simulink model "PMSM_New_MTPA"  (R2018b)
settings: Solver=ode45  StartTime=0.0  StopTime=15  FixedStep=Ts  RelTol=1e-4  EnableMultiTasking=on
InitFcn:
  | Ts = 1e-4;
  | 
  | 
  | Rs = 0.8975;
  | Ld = 15e-3;
  | Lq = 19e-3;
  | Pn = 3;
  | flux = 0.1764;
  | 
  | kp_comp = 0.65;
  | ki_comp = 0.001*pi*kp_comp;
  | 
  | kp_FW = 1;
  | ki_FW = 0;
undefined symbols (not defined in the file or in its folder): DiscIntNeverNeededParam
libraries: powerlib x5, powerlib_extras x2, simulink x1
settings Model: Creator=SUN  LastModifiedBy=liangjin
settings SolverCC: ZeroCrossControl=DisableAll
settings DataIOCC: LimitDataPoints=on  SaveFormat=Array
settings OptimizationCC: ExpressionDepthLimit=2147483647  InitFltsAndDblsToZero=on  LifeSpan=inf
settings DebuggingCC: UnderspecifiedInitializationDetection=Classic  MergeDetectMultiDrivingBlocksExec=none  SolverPrmCheckMsg=warning  FcnCallInpInsideContextMsg=warning  StateNameClashWarn=warning  SFUnexpectedBacktrackingDiag=warning  SFNoUnconditionalDefaultTransitionDiag=warning  SFExecutionAtInitializationDiag=none
settings HardwareCC: ProdBitPerPointer=32  ProdBitPerSizeT=32  ProdBitPerPtrDiffT=32  ProdLargestAtomicFloat=None  ProdIntDivRoundTo=Undefined  ProdEndianess=Unspecified  ProdWordSize=32  ProdHWDeviceType=32-bit Generic
settings ModelReferenceCC: PropagateSignalLabelsOutOfModel=off
settings SFSimCC: SimUseLocalCustomCode=off
settings RTWCC: RTWUseLocalCustomCode=off
settings CodeAppCC: StateflowObjectComments=on
settings GRTTargetCC: TargetLangStandard=C89/C90 (ANSI)  GeneratePreprocessorConditionals=Disable all  CombineOutputUpdateFcns=off  GRTInterface=on
settings ConfigComp: CovMetricSettings=dw  CovHtmlReporting=on  CovSaveCumulativeToWorkspaceVar=on  CovSaveSingleToWorkspaceVar=on  CovExternalEMLEnable=off  CovSFcnEnable=off
settings SimscapeCC: SimscapeNormalizeSystem=off

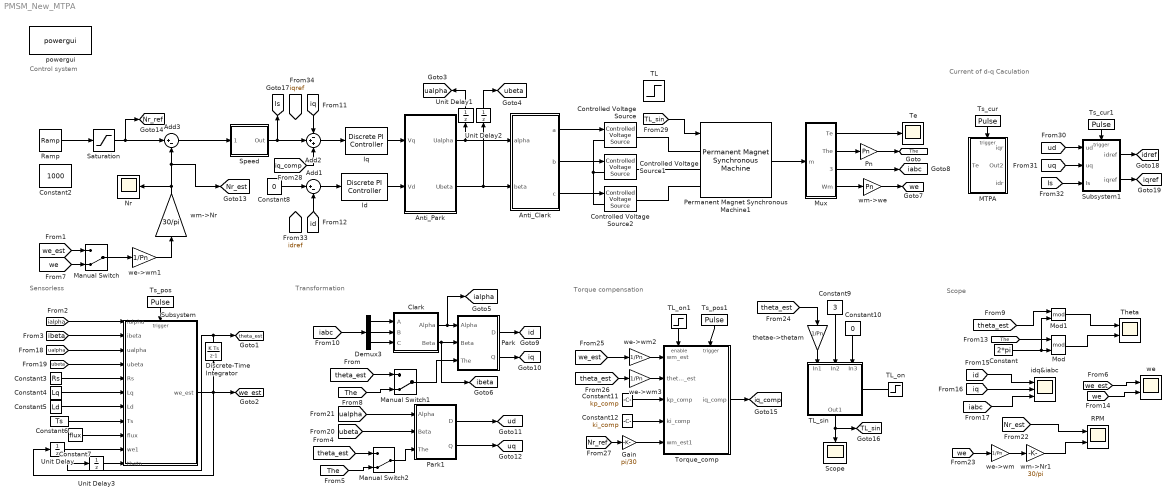
== system PMSM_New_MTPA ==
  note: Torque compensation
  note: Scope
  note: Control system
  note: Transformation
  note: Sensorless
  note: Current of d-q Caculation
  Add1 : Sum  Inputs=|+-
  Add2 : Sum  Inputs=-++
  Add3 : Sum  Inputs=|+-
  Anti_Clark : Subsystem
  Anti_Park : Subsystem
  Clark : Subsystem
  Constant : Constant  Value=2*pi
  Constant10 : Constant  Value=0
  Constant11 : Constant  Value=kp_comp
  Constant12 : Constant  Value=ki_comp
  Constant2 : Constant  Value=1000
  Constant3 : Constant  Value=Rs
  Constant4 : Constant  Value=Lq
  Constant5 : Constant  Value=Ld
  Constant6 : Constant  Value=Ts
  Constant7 : Constant  Value=flux
  Constant8 : Constant  Value=0
  Constant9 : Constant  Value=3
  Controlled Voltage Source : powerlib/Electrical Sources/Controlled Voltage Source  Initialize=on  Source_Type=AC  Amplitude=0  Phase=0  Frequency=0  Measurements=Voltage
      settings: SourceProductName=Simscape Electrical
  Controlled Voltage Source1 : powerlib/Electrical Sources/Controlled Voltage Source  Initialize=on  Source_Type=AC  Amplitude=0  Phase=0  Frequency=0  Measurements=Voltage
      settings: SourceProductName=Simscape Electrical
  Controlled Voltage Source2 : powerlib/Electrical Sources/Controlled Voltage Source  Initialize=on  Source_Type=AC  Amplitude=0  Phase=0  Frequency=0  Measurements=Voltage
      settings: SourceProductName=Simscape Electrical
  Demux3 : Demux  Outputs=3
  Discrete-Time Integrator : DiscreteIntegrator  gainval=1  SampleTime=Ts  ICPrevOutput=DiscIntNeverNeededParam  ICPrevScaledInput=DiscIntNeverNeededParam
  Gain : Gain  Gain=pi/30
  Id : powerlib_extras/Discrete  Control Blocks/Discrete PI Controller  Kp=Ld*376  Ki=Rs*376  Par_Limits=[311*sqrt(1/3) -311*sqrt(1/3)]  Init=0  Ts=Ts
  Iq : powerlib_extras/Discrete  Control Blocks/Discrete PI Controller  Kp=Lq*376  Ki=Rs*376  Par_Limits=[311*sqrt(1/3) -311*sqrt(1/3)]  Init=0  Ts=Ts
  MTPA : Subsystem
  Manual Switch : ManualSwitch  CurrentSetting=0
  Manual Switch1 : ManualSwitch  CurrentSetting=0
  Manual Switch2 : ManualSwitch  CurrentSetting=0
  Mod : Math  Operator=mod  SaturateOnIntegerOverflow=on
  Mod1 : Math  Operator=mod  SaturateOnIntegerOverflow=on
  Mux : Subsystem
  Nr : Scope
  Park : Subsystem
  Park1 : Subsystem
  Permanent Magnet Synchronous Machine1 : powerlib/Machines/Permanent Magnet Synchronous Machine  NbPhases=3  FluxDistribution=Sinusoidal  RotorType=Salient-pole  MechanicalLoad=Torque Tm  PresetModel=No  ShowDetailedParameters=on  MeasurementBus=off  Resistance=0.8975  Inductance=8.5e-3  dqInductances=[15e-3,19e-3]  La=0.000835  MachineConstant=Flux linkage established by magnets (V.s)  Flux=0.1764  VoltageCst=95.9863  TorqueCst=0.7938  Flat=120  Mechanical=[0.000311 0.0000001 3]  PolePairs=3  InitialConditions=[0,0, 0,0]  InitialConditions5ph=[0 0 0 0 0 0]  TsPowergui=0  TsBlock=Ts  RefAngle=Aligned with phase A axis (original Park)
  Pn : Gain  Gain=Pn
  RPM : Scope  NumInputPorts=2
  Ramp : simulink/Sources/Ramp  slope=250  start=0  InitialOutput=0
  Saturation : Saturate  UpperLimit=1000  LowerLimit=-1000
  Scope : Scope
  Speed : Subsystem  AncestorBlock=|  DialogController=POWERSYS.PowerSysDialog  mask(Discrete PI Controller){Kpw=0.01, Kiw=0.01*50, Ba=0, Par_Limits=[50 -50], Init=0, Ts=Ts}
      | powerlib_extras/Discrete 
      | Control Blocks/Discrete
      | PI Controller
      mask prompts: Kpw "Proportional gain (Kp):"; Kiw "Integral gain (Ki):"; Ba "feedback gain (Ba)"; Par_Limits "Output limits: [ Upper   Lower ]"; Init "Output initial value:"; Ts "Sample time:"
      mask help: This block implements a discrete PI controller.
      mask init:
      | UpperLimit=Par_Limits(1);
      | LowerLimit=Par_Limits(2);
      | power_initmask();
      mask Help: This block is part of a subset of blocks in the Extras library that does not have documentation associated with it, other than the block mask description.
      mask Display: disp('PI');
  Subsystem : Subsystem
  Subsystem1 : Subsystem
  TL : Step  Time=5  After=7  SampleTime=Ts
  TL_on : Step  Time=5  SampleTime=0
  TL_on1 : Step  Time=5  SampleTime=0
  TL_sin : Subsystem
  Te : Scope
  Theta : Scope  NumInputPorts=2
  Torque_comp : Subsystem
  Ts_cur : DiscretePulseGenerator  PulseType=Time based  Period=Ts  PulseWidth=50
  Ts_cur1 : DiscretePulseGenerator  PulseType=Time based  Period=Ts  PulseWidth=50
  Ts_pos : DiscretePulseGenerator  PulseType=Time based  Period=Ts  PulseWidth=50
  Ts_pos1 : DiscretePulseGenerator  PulseType=Time based  Period=Ts  PulseWidth=50
  Unit Delay{,1..3} (4 alike) : UnitDelay  SampleTime=Ts
  idq&iabc : Scope  NumInputPorts=3
  powergui : powerlib/powergui  SimulationMode=Discrete  SampleTime=1e-5  frequency=60  Iterations=50  frequencyindice=0  Pbase=100e6  ErrMax=1e-4  UnitsV=kV  UnitsW=MW  buscounter=0  FunctionMessages=off  echomessages=off  EnableUseOfTLC=off  CurrentSourceSwitches=off  DisableSnubberDevices=off  DisableRonSwitches=off  DisableVfSwitches=off  DisplayEquations=off  SolverType=Tustin/Backward Euler (TBE)  Interpol=off  ExternalGateDelay=off  methode=off  Ts=100  x0status=blocks  SPID=off  SwTol=0  HookPort=off  RestoreLinks=warning  ResistiveCurrentMeasurement=off  Frange=[0:2:500]  Ylog=off  Xlog=on  ShowGrid=off  save=off  variable=ZData  structure=0  ZoomFFT=on  StartTime=0.0  cycles=1  DisplayStyle=1  fundamental=60  FreqAxis=off  MaxFrequency=1000  frequencyindicesteady=1  RmsSteady=1  display=off
  thetae->thetam : Gain  Gain=1/Pn
  we : Scope  NumInputPorts=2
  we->wm{,1..3} (4 alike) : Gain  Gain=1/Pn
  wm->Nr : Gain  Gain=30/pi
  wm->Nr1 : Gain  Gain=30/pi
  wm->we : Gain  Gain=Pn
  tag scope: Is=global, Nr_est=global, Nr_ref=global, TL_sin=global, The=global, iabc=global, ialpha=global, ibeta=global, id=global, idref=global, iq=global, iq_comp=global, iqref=global, theta_est=global, ualpha=global, ubeta=global, ud=global, uq=global, we=global, we_est=global
  wires:
  Permanent Magnet Synchronous Machine1/1 -> Mux/1(m)
  Add3/1 -> Speed/1(Error)
  wm->Nr/1 -> [Nr_est], Add3/2, Nr/1
  Mux/1(Te) -> Te/1
  Mux/2(The) -> Pn/1
  Pn/1 -> [The]
  Mux/4(Wm) -> wm->we/1
  Mux/3(Iabc) -> [iabc]
  Clark/1(Alpha) -> [ialpha], Park/1(Alpha)
  Demux3/1 -> Clark/1(A)
  Demux3/2 -> Clark/2(B)
  Demux3/3 -> Clark/3(C)
  Clark/2(Beta) -> Park/2(Beta), [ibeta]
  Iq/1 -> Anti_Park/1(Vq)
  Id/1 -> Anti_Park/2(Vd)
  Anti_Clark/2(b) -> Controlled Voltage Source1/1
  Anti_Clark/3(c) -> Controlled Voltage Source2/1
  Constant/1 -> Mod1/2, Mod/2
  Mod/1 -> Theta/2
  wm->we/1 -> [we]
  Ramp/1 -> Saturation/1
  we->wm1/1 -> wm->Nr/1
  Anti_Park/1(Ualpha) -> Unit Delay1/1, Anti_Clark/1(alpha)
  Anti_Park/2(Ubeta) -> Unit Delay2/1, Anti_Clark/2(beta)
  [we_est] -> we/1
  [we_est] -> Manual Switch/1
  [we] -> Manual Switch/2
  [theta_est] -> Manual Switch1/1
  Manual Switch1/1 -> Park/3(The)
  [The] -> Manual Switch1/2
  Park/1(D) -> [id]
  Park/2(Q) -> [iq]
  [The] -> Mod/1
  [id] -> idq&iabc/1
  [iq] -> idq&iabc/2
  [iabc] -> idq&iabc/3
  [id] -> Add1/2
  [iq] -> Add2/1
  Manual Switch/1 -> we->wm1/1
  [The] -> Manual Switch2/2
  Manual Switch2/1 -> Park1/3(The)
  [theta_est] -> Manual Switch2/1
  [ubeta] -> Park1/2(Beta)
  [ualpha] -> Park1/1(Alpha)
  Park1/1(D) -> [ud]
  Park1/2(Q) -> [uq]
  Unit Delay1/1 -> [ualpha]
  Unit Delay2/1 -> [ubeta]
  Subsystem/1(we_est) -> Discrete-Time Integrator/1, [we_est], Unit Delay/1
  Constant3/1 -> Subsystem/5(Rs)
  Constant4/1 -> Subsystem/6(Lq)
  Constant5/1 -> Subsystem/7(Ld)
  Constant6/1 -> Subsystem/8(Ts)
  Constant7/1 -> Subsystem/9(flux)
  Unit Delay/1 -> Subsystem/10(we1)
  Ts_pos/1 -> Subsystem/Trigger
  Unit Delay3/1 -> Subsystem/11(theta)
  [theta_est] -> Mod1/1
  Mod1/1 -> Theta/1
  [iabc] -> Demux3/1
  Discrete-Time Integrator/1 -> [theta_est], Unit Delay3/1
  Anti_Clark/1(a) -> Controlled Voltage Source/1
  [ialpha] -> Subsystem/1(ialpha)
  [ibeta] -> Subsystem/2(ibeta)
  [ualpha] -> Subsystem/3(ualpha)
  [ubeta] -> Subsystem/4(ubeta)
  [we] -> we->wm/1
  we->wm/1 -> wm->Nr1/1
  wm->Nr1/1 -> RPM/2
  [Nr_est] -> RPM/1
  Saturation/1 -> [Nr_ref], Add3/1
  Ts_cur/1 -> MTPA/Trigger
  Add2/1 -> Iq/1
  Add1/1 -> Id/1
  [we] -> we/2
  [theta_est] -> thetae->thetam/1
  thetae->thetam/1 -> TL_sin/1(In1)
  Constant9/1 -> TL_sin/2(In2)
  Constant10/1 -> TL_sin/3(In3)
  TL_on/1 -> TL_sin/Enable
  Speed/1(Out) -> Add2/2, [Is]
  TL_sin/1(Out1) -> [TL_sin], Scope/1
  we->wm2/1 -> Torque_comp/1(wm_est)
  we->wm3/1 -> Torque_comp/2(thetam_est)
  Constant11/1 -> Torque_comp/3(kp_comp)
  Constant12/1 -> Torque_comp/4(ki_comp)
  Torque_comp/1(iq_comp) -> [iq_comp]
  [Nr_ref] -> Gain/1
  Gain/1 -> Torque_comp/5(wm_est1)
  Ts_pos1/1 -> Torque_comp/Trigger
  TL_on1/1 -> Torque_comp/Enable
  [we_est] -> we->wm2/1
  [theta_est] -> we->wm3/1
  [ud] -> Subsystem1/1(ud)
  [uq] -> Subsystem1/2(uq)
  [Is] -> Subsystem1/3(Is)
  Ts_cur1/1 -> Subsystem1/Trigger
  Subsystem1/1(idref) -> [idref]
  Subsystem1/2(iqref) -> [iqref]
  Constant8/1 -> Add1/1
  [iq_comp] -> Add2/3
  [TL_sin] -> Permanent Magnet Synchronous Machine1/1
  connections:
  Controlled Voltage Source/LConn1 -- Controlled Voltage Source2/LConn1 -- Controlled Voltage Source1/LConn1
  Controlled Voltage Source/RConn1 -- Permanent Magnet Synchronous Machine1/LConn1
  Controlled Voltage Source1/RConn1 -- Permanent Magnet Synchronous Machine1/LConn2
  Controlled Voltage Source2/RConn1 -- Permanent Magnet Synchronous Machine1/LConn3

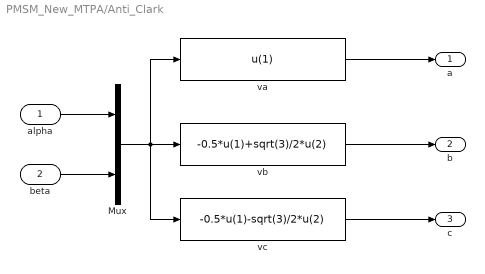
== system PMSM_New_MTPA/Anti_Clark ==
  alpha : Inport
  beta : Inport  Port=2
  Mux : Mux  Inputs=2
  va : Fcn  Expr=u(1)
  vb : Fcn  Expr=-0.5*u(1)+sqrt(3)/2*u(2)
  vc : Fcn  Expr=-0.5*u(1)-sqrt(3)/2*u(2)
  a : Outport
  b : Outport  Port=2
  c : Outport  Port=3
  wires:
  va/1 -> a/1
  beta/1 -> Mux/2
  alpha/1 -> Mux/1
  Mux/1 -> vc/1, vb/1, va/1
  vb/1 -> b/1
  vc/1 -> c/1

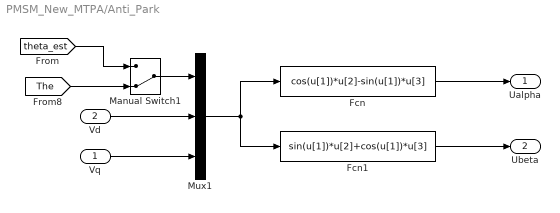
== system PMSM_New_MTPA/Anti_Park ==
  Vq : Inport
  Vd : Inport  Port=2
  Fcn : Fcn  Expr=cos(u[1])*u[2]-sin(u[1])*u[3]
  Fcn1 : Fcn  Expr=sin(u[1])*u[2]+cos(u[1])*u[3]
  Manual Switch1 : ManualSwitch  CurrentSetting=0
  Mux1 : Mux  Inputs=3
  Ualpha : Outport
  Ubeta : Outport  Port=2
  wires:
  Fcn1/1 -> Ubeta/1
  Fcn/1 -> Ualpha/1
  Mux1/1 -> Fcn/1, Fcn1/1
  Vd/1 -> Mux1/2
  Vq/1 -> Mux1/3
  Manual Switch1/1 -> Mux1/1
  [The] -> Manual Switch1/2
  [theta_est] -> Manual Switch1/1

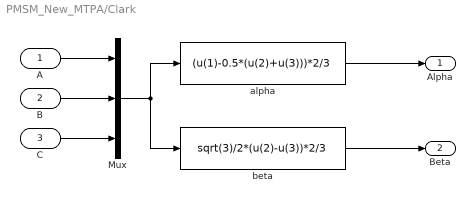
== system PMSM_New_MTPA/Clark ==
  A : Inport
  B : Inport  Port=2
  C : Inport  Port=3
  Mux : Mux  Inputs=3
  alpha : Fcn  Expr=(u(1)-0.5*(u(2)+u(3)))*2/3
  beta : Fcn  Expr=sqrt(3)/2*(u(2)-u(3))*2/3
  Alpha : Outport
  Beta : Outport  Port=2
  wires:
  alpha/1 -> Alpha/1
  B/1 -> Mux/2
  C/1 -> Mux/3
  A/1 -> Mux/1
  Mux/1 -> beta/1, alpha/1
  beta/1 -> Beta/1

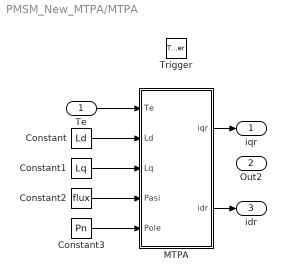
== system PMSM_New_MTPA/MTPA ==
  Te : Inport
  Trigger : TriggerPort  VariantControl=Variant  PortDimensions=1
  Constant : Constant  Value=Ld
  Constant1 : Constant  Value=Lq
  Constant2 : Constant  Value=flux
  Constant3 : Constant  Value=Pn
  MTPA : MATLAB Function  TreatAsAtomicUnit=on
  iqr : Outport
  Out2 : Outport  Port=2
  idr : Outport  Port=3
  wires:
  MTPA/2(idr) -> idr/1
  MTPA/1(iqr) -> iqr/1
  Te/1 -> MTPA/1(Te)
  Constant/1 -> MTPA/2(Ld)
  Constant1/1 -> MTPA/3(Lq)
  Constant3/1 -> MTPA/5(Pole)
  Constant2/1 -> MTPA/4(Pasi)

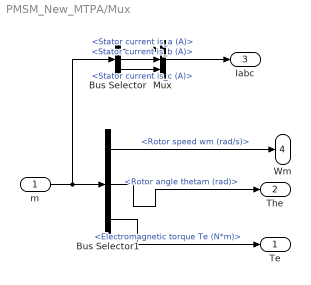
== system PMSM_New_MTPA/Mux ==
  m : Inport
  Bus Selector : BusSelector  OutputSignals=Stator current is_a (A),Stator current is_b (A),Stator current is_c (A)
  Bus Selector1 : BusSelector  OutputSignals=Rotor speed wm (rad/s),Rotor angle thetam (rad),Electromagnetic torque Te (N*m)
  Mux : Mux  Inputs=3
  Te : Outport
  The : Outport  Port=2
  Iabc : Outport  Port=3
  Wm : Outport  Port=4
  wires:
  Bus Selector1/1 -> Wm/1  "<Rotor speed wm (rad/s)>"
  Bus Selector1/2 -> The/1  "<Rotor angle thetam (rad)>"
  Bus Selector1/3 -> Te/1  "<Electromagnetic torque Te (N*m)>"
  m/1 -> Bus Selector/1, Bus Selector1/1
  Bus Selector/2 -> Mux/2  "<Stator current is_b (A)>"
  Bus Selector/3 -> Mux/3  "<Stator current is_c (A)>"
  Bus Selector/1 -> Mux/1  "<Stator current is_a (A)>"
  Mux/1 -> Iabc/1

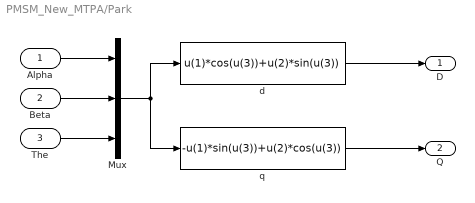
== system PMSM_New_MTPA/Park ==
  Alpha : Inport
  Beta : Inport  Port=2
  The : Inport  Port=3
  Mux : Mux  Inputs=3
  d : Fcn  Expr=u(1)*cos(u(3))+u(2)*sin(u(3))
  q : Fcn  Expr=-u(1)*sin(u(3))+u(2)*cos(u(3))
  D : Outport
  Q : Outport  Port=2
  wires:
  d/1 -> D/1
  Beta/1 -> Mux/2
  Alpha/1 -> Mux/1
  Mux/1 -> q/1, d/1
  q/1 -> Q/1
  The/1 -> Mux/3

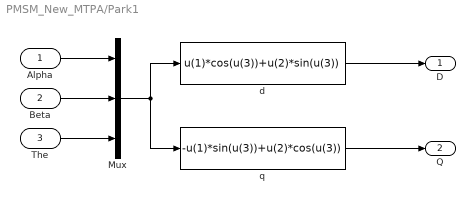
== system PMSM_New_MTPA/Park1 ==
  Alpha : Inport
  Beta : Inport  Port=2
  The : Inport  Port=3
  Mux : Mux  Inputs=3
  d : Fcn  Expr=u(1)*cos(u(3))+u(2)*sin(u(3))
  q : Fcn  Expr=-u(1)*sin(u(3))+u(2)*cos(u(3))
  D : Outport
  Q : Outport  Port=2
  wires:
  d/1 -> D/1
  Beta/1 -> Mux/2
  Alpha/1 -> Mux/1
  Mux/1 -> q/1, d/1
  q/1 -> Q/1
  The/1 -> Mux/3

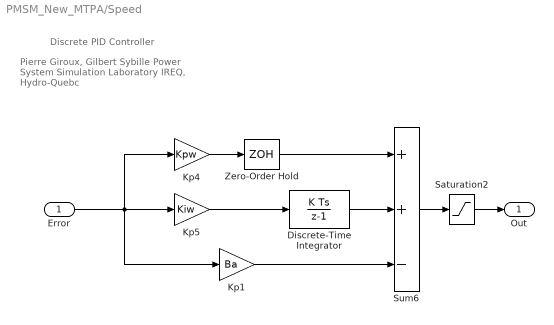
== system PMSM_New_MTPA/Speed ==
  note: Discrete PID Controller
  note: Pierre Giroux, Gilbert Sybille
      | Power System Simulation Laboratory
      | IREQ, Hydro-Quebc
  Error : Inport  SampleTime=Ts
  Discrete-Time Integrator : DiscreteIntegrator  InitialCondition=Init  SampleTime=Ts  LimitOutput=on  UpperSaturationLimit=UpperLimit  LowerSaturationLimit=LowerLimit  ICPrevOutput=DiscIntNeverNeededParam  ICPrevScaledInput=DiscIntNeverNeededParam
  Kp1 : Gain  Gain=Ba  SampleTime=Ts  SaturateOnIntegerOverflow=on  OutDataTypeStr=Inherit: Same as input  ParamDataTypeStr=Inherit: Same as input
  Kp4 : Gain  Gain=Kpw  SampleTime=Ts  SaturateOnIntegerOverflow=on  OutDataTypeStr=Inherit: Same as input  ParamDataTypeStr=Inherit: Same as input
  Kp5 : Gain  Gain=Kiw  SampleTime=Ts  SaturateOnIntegerOverflow=on  OutDataTypeStr=Inherit: Same as input  ParamDataTypeStr=Inherit: Same as input
  Saturation2 : Saturate  UpperLimit=UpperLimit  LowerLimit=LowerLimit  SampleTime=Ts
  Sum6 : Sum  Inputs=++-  SampleTime=Ts  SaturateOnIntegerOverflow=on  InputSameDT=on  OutDataTypeStr=Inherit: Same as first input
  Zero-Order Hold : ZeroOrderHold  SampleTime=Ts
  Out : Outport  SampleTime=Ts  InitialOutput=0
  wires:
  Error/1 -> Kp1/1, Kp5/1, Kp4/1
  Zero-Order Hold/1 -> Sum6/1
  Saturation2/1 -> Out/1
  Discrete-Time Integrator/1 -> Sum6/2
  Kp4/1 -> Zero-Order Hold/1
  Kp5/1 -> Discrete-Time Integrator/1
  Sum6/1 -> Saturation2/1
  Kp1/1 -> Sum6/3

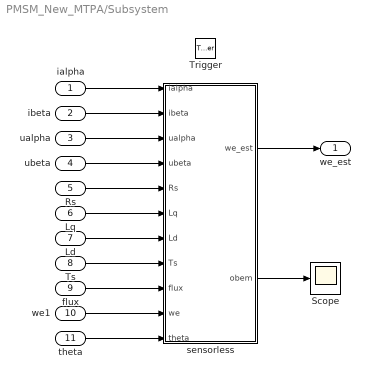
== system PMSM_New_MTPA/Subsystem ==
  ialpha : Inport
  ibeta : Inport  Port=2
  ualpha : Inport  Port=3
  ubeta : Inport  Port=4
  Rs : Inport  Port=5
  Lq : Inport  Port=6
  Ld : Inport  Port=7
  Ts : Inport  Port=8
  flux : Inport  Port=9
  we1 : Inport  Port=10
  theta : Inport  Port=11
  Trigger : TriggerPort  VariantControl=Variant  PortDimensions=1
  Scope : Scope
  sensorless : MATLAB Function  TreatAsAtomicUnit=on
  we_est : Outport
  wires:
  ualpha/1 -> sensorless/3(ualpha)
  Ts/1 -> sensorless/8(Ts)
  flux/1 -> sensorless/9(flux)
  ialpha/1 -> sensorless/1(ialpha)
  sensorless/1(we_est) -> we_est/1
  Lq/1 -> sensorless/6(Lq)
  ubeta/1 -> sensorless/4(ubeta)
  ibeta/1 -> sensorless/2(ibeta)
  Rs/1 -> sensorless/5(Rs)
  Ld/1 -> sensorless/7(Ld)
  we1/1 -> sensorless/10(we)
  theta/1 -> sensorless/11(theta)
  sensorless/2(obem) -> Scope/1

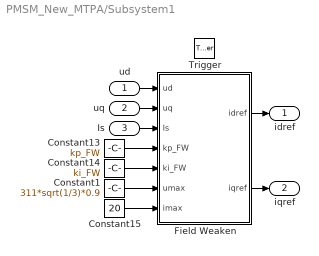
== system PMSM_New_MTPA/Subsystem1 ==
  ud : Inport
  uq : Inport  Port=2
  Is : Inport  Port=3
  Trigger : TriggerPort  VariantControl=Variant  PortDimensions=1
  Constant1 : Constant  Value=311*sqrt(1/3)*0.9
  Constant13 : Constant  Value=kp_FW
  Constant14 : Constant  Value=ki_FW
  Constant15 : Constant  Value=20
  Field Weaken : MATLAB Function  TreatAsAtomicUnit=on
  idref : Outport
  iqref : Outport  Port=2
  wires:
  Constant13/1 -> Field Weaken/4(kp_FW)
  Constant15/1 -> Field Weaken/7(imax)
  Field Weaken/1(idref) -> idref/1
  Constant14/1 -> Field Weaken/5(ki_FW)
  uq/1 -> Field Weaken/2(uq)
  Constant1/1 -> Field Weaken/6(umax)
  Field Weaken/2(iqref) -> iqref/1
  ud/1 -> Field Weaken/1(ud)
  Is/1 -> Field Weaken/3(Is)

== system PMSM_New_MTPA/TL_sin ==
  In1 : Inport
  In2 : Inport  Port=2
  In3 : Inport  Port=3
  Enable : EnablePort
  MATLAB Function : MATLAB Function  TreatAsAtomicUnit=on
  Out1 : Outport
  wires:
  In1/1 -> MATLAB Function/1(Theta_m)
  MATLAB Function/1(TL) -> Out1/1
  In3/1 -> MATLAB Function/3(Theta0)
  In2/1 -> MATLAB Function/2(Amp)

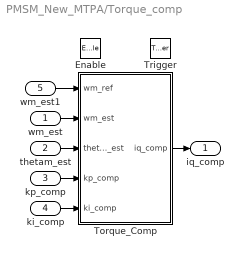
== system PMSM_New_MTPA/Torque_comp ==
  wm_est : Inport
  thetam_est : Inport  Port=2
  kp_comp : Inport  Port=3
  ki_comp : Inport  Port=4
  wm_est1 : Inport  Port=5
  Enable : EnablePort
  Trigger : TriggerPort  VariantControl=Variant  PortDimensions=1
  Torque_Comp : MATLAB Function  TreatAsAtomicUnit=on
  iq_comp : Outport
  wires:
  Torque_Comp/1(iq_comp) -> iq_comp/1
  kp_comp/1 -> Torque_Comp/4(kp_comp)
  wm_est/1 -> Torque_Comp/2(wm_est)
  ki_comp/1 -> Torque_Comp/5(ki_comp)
  wm_est1/1 -> Torque_Comp/1(wm_ref)
  thetam_est/1 -> Torque_Comp/3(thetam_est)

== matlab function PMSM_New_MTPA/MTPA/MTPA ==
  data: iqr output; Te input; idr output; Ld input; Lq input; Pasi input; Pole input
function [iqr,idr] = MTPA(Te,Ld,Lq,Pasi,Pole)

persistent id1 iq1 temp1 temp2 temp3;

if isempty(id1)
    id1=0;iq1=0;temp1=0;temp2=0;temp3 = 0;
end
temp1 = Pasi.^2 - 4*(Ld-Lq).^2;
temp2 = 8*Te*Pasi/(3*Pole);
temp3 = temp2.^2-4*temp1*((4*Te/3/Pole).^2-Pasi.^2);

if (temp3 < 0)
    temp3 = 0;
end

iq1 = (temp2 + sqrt(temp3))/(2*temp1);
id1 = Pasi/(2*Lq-2*Ld) - sqrt((Pasi/(2*Lq-2*Ld)).^2+iq1.^2);

idr = id1;
iqr = iq1;

== matlab function PMSM_New_MTPA/Subsystem/sensorless ==
  data: ialpha input; we_est output; ibeta input; ualpha input; ubeta input; Rs input; Lq input; Ld input; Ts input; flux input; we input; theta input; obem output

function [we_est, obem]  = sensorless(ialpha,ibeta,ualpha,ubeta,Rs,Lq,Ld,Ts,flux,we,theta)

persistent id2 iq2 delta_id delta_iq bemf we1 flag;

if isempty(id2)
    id2=0;iq2=0;delta_id=0;delta_iq=0;bemf=0;we1=0;flag=0;obem=0;
end

ud= cos(theta)*ualpha+sin(theta)*ubeta;
uq=-sin(theta)*ualpha+cos(theta)*ubeta;
id1= cos(theta)*ialpha+sin(theta)*ibeta;
iq1=-sin(theta)*ialpha+cos(theta)*ibeta;

if(bemf < 0)
    flag = 1;
end

we1 = we1+0.715*(we-we1);
temp1 = ud-id2*Rs;
temp1 = temp1+we1*Lq*iq2;
temp1 = temp1*Ts/Ld + id2;
delta_id = delta_id+0.125*((temp1-id1)-delta_id);

temp2 = uq-iq2*Rs;
temp2 = temp2-we1*Ld*id2;
temp2 = temp2-bemf;
temp2 = Ts*temp2/Lq+iq2;
delta_iq = delta_iq+0.5*((temp2-iq1)-delta_iq);

bemf = bemf+delta_iq*Lq/Ts;
if(flag)
    we_est = (bemf+delta_id*Ld/Ts)/flux;
else
    we_est = (bemf-delta_id*Ld/Ts)/flux;
end
obem = bemf;
id2 = id1;
iq2 = iq1;

== matlab function PMSM_New_MTPA/TL_sin/MATLAB Function ==
  data: Theta_m input; TL output; Amp input; Theta0 input
function TL = fcn(Theta_m,Amp,Theta0)
if isempty(Theta_m)
    Theta_m=0;Amp=0;Theta0=0;TL=0;
end
TL = Amp*sin(Theta_m+Theta0);

== matlab function PMSM_New_MTPA/Torque_comp/Torque_Comp ==
  data: wm_ref input; iq_comp output; wm_est input; thetam_est input; kp_comp input; ki_comp input
function iq_comp = Torque_Comp(wm_ref,wm_est,thetam_est,kp_comp,ki_comp)

persistent Te temp1 temp2 up ui1 ui2 out1 out2 comp1_fbk comp2_fbk comp1_ref comp2_ref;

if isempty(temp1)
    Te=0; temp1=0; temp2=0; up=0; ui1=0; ui2=0; out1=0; out2=0; iq_comp=0; 
    comp1_fbk=0; comp2_fbk=0; comp1_ref=0; comp2_ref=0;
end

%calc comp sin value
Te = wm_ref-wm_est;
temp1 = Te*sin(thetam_est);
comp1_fbk = 0;
if (wm_ref < 10)
    comp1_ref = 0;
else
    comp1_ref = temp1;
end
up = comp1_ref - comp1_fbk;
ui1 = ui1 + ki_comp*up;
out1 = kp_comp*up + ui1;

%calc comp cos value
temp2 = Te*cos(thetam_est);
comp2_fbk = 0;
if (wm_ref < 10)
    comp2_ref = 0;
else
    comp2_ref = temp2;
end
up = comp2_ref - comp2_fbk;
ui2 = ui2 + ki_comp*up;
out2 = kp_comp*up + ui2;

iq_comp = out1*sin(thetam_est) + out2*cos(thetam_est);

if (iq_comp > 10)
    iq_comp = 10;
elseif (iq_comp < -10)
    iq_comp = -10;
end

== matlab function PMSM_New_MTPA/Subsystem1/Field Weaken ==
  data: idref output; iqref output; ud input; uq input; Is input; kp_FW input; ki_FW input; umax input; imax input
function [idref,iqref] = Fieldweaken(ud,uq,Is,kp_FW,ki_FW,umax,imax)

persistent us gama uout ui temp id1 iq1;

isempty (us)
us=0;gama=0;ui=0;temp=0;uout=0;id1=0;iq1=0;

us = sqrt(ud.^2+uq.^2);
if(us<umax)
    id1 = 0; iq1 = Is;
elseif(us>=umax)
    temp = us - umax;
    ui = ui + temp;
    uout = kp_FW*temp+ki_FW*ui;
    if(uout>=0)
        uout = 0;
    elseif(uout<=-pi/2)
        uout = -pi/2;
    end
    gama = uout;
    iq1 = Is*cos(gama);
    id1 = Is*sin(gama);
end

if (id1<-imax)
    id1 = -imax;
end

idref = id1;
iqref = iq1;
